simulink model "PMSM_SVPWM"  (R2021b)
settings: Solver=ode23tb  StartTime=0.0  StopTime=1  RelTol=1e-3  EnableMultiTasking=on
InitFcn:
  | flux=0.192;
  | Ld=0.0006033;
  | Lq=0.0006668;
  | R=0.05;
libraries: powerlib_extras x3, spsDCVoltageSourceLib x1, eeTransforms x1, spsPermanentMagnetSynchronousMachineLib x1, simulink x1, spsUniversalBridgeLib x1, spsVoltageMeasurementLib x1, spsdq0toabcLib x1, spspowerguiLib x1
settings Model: Creator=LZ  LastModifiedBy=wkw
settings SolverCC: AlgebraicLoopSolver=TrustRegion
settings DataIOCC: LimitDataPoints=on  SaveFormat=Array  ReturnWorkspaceOutputs=off
settings OptimizationCC: EfficientMapNaN2IntZero=off  LifeSpan=inf
settings DebuggingCC: SolverPrmCheckMsg=warning  SFUnexpectedBacktrackingDiag=warning  SFNoUnconditionalDefaultTransitionDiag=warning  SFMachineParentedDataDiag=warning  ArithmeticOperatorsInVariantConditions=warning
settings HardwareCC: ProdBitPerPointer=32  ProdBitPerSizeT=32  ProdBitPerPtrDiffT=32  ProdLargestAtomicFloat=None  ProdIntDivRoundTo=Undefined  ProdEndianess=Unspecified  ProdWordSize=32  ProdHWDeviceType=32-bit Generic  TargetBitPerLong=64  TargetBitPerPointer=64  TargetBitPerSizeT=64  TargetBitPerPtrDiffT=64  TargetLongLongMode=on  TargetIntDivRoundTo=Zero  TargetEndianess=LittleEndian  TargetWordSize=64  TargetHWDeviceType=MATLAB Host  ProdEqTarget=off
settings ModelReferenceCC: PropagateSignalLabelsOutOfModel=off
settings SFSimCC: SimUseLocalCustomCode=off  CustomCodeUndefinedFunction=UseInterfaceOnly
settings RTWCC: RTWUseLocalCustomCode=off
settings CodeAppCC: MaxIdLength=128  StateflowObjectComments=on
settings GRTTargetCC: TargetLangStandard=C89/C90 (ANSI)  CombineOutputUpdateFcns=off  GRTInterface=on
settings ConfigComp: CovMetricSettings=dw  CovSaveCumulativeToWorkspaceVar=on  CovSaveSingleToWorkspaceVar=on  CovExternalEMLEnable=off  CovSFcnEnable=off
settings SimscapeCC: SimscapeNormalizeSystem=off

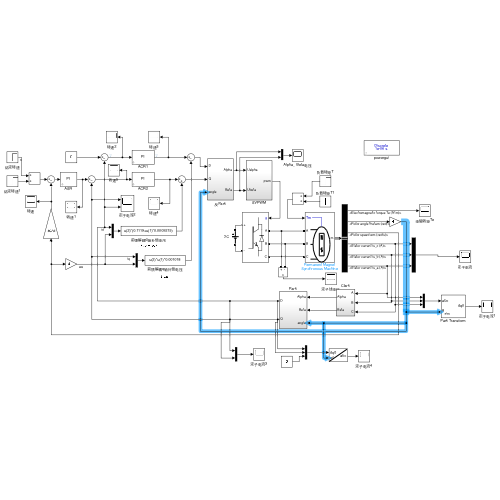
[thumbnail: Simulink's stored preview of the top-level diagram]
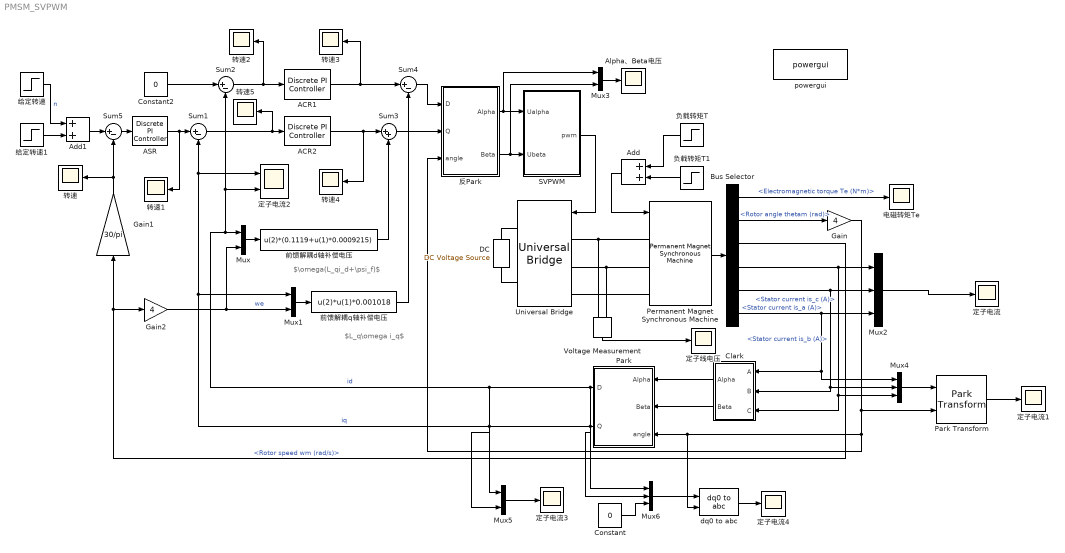
== system PMSM_SVPWM ==
  note: $\omega(L_qi_d+\psi_f)$
  note: $L_q\omega i_q$
  ACR1 : powerlib_extras/Discrete  Control Blocks/Discrete PI Controller  Kp=4  Ki=80  Par_Limits=[560*0.9*sqrt(1/3) -560*0.9*sqrt(1/3)]  Init=0  Ts=1e-6
  ACR2 : powerlib_extras/Discrete  Control Blocks/Discrete PI Controller  Kp=4  Ki=80  Par_Limits=[560*0.9*sqrt(1/3) -560*0.9*sqrt(1/3)]  Init=0  Ts=1e-6
  ASR : powerlib_extras/Discrete  Control Blocks/Discrete PI Controller  Kp=5  Ki=200  Par_Limits=[65 -65]  Init=0  Ts=1e-6
  Add : Sum
  Add1 : Sum
  Alpha、Beta电压 : Scope
  Bus Selector : BusSelector  OutputSignals=Electromagnetic torque Te (N*m),Rotor angle thetam (rad),Rotor speed wm (rad/s),Stator current is_c (A),Stator current is_b (A),Stator current is_a (A)
  Clark : Subsystem
  Constant : Constant  Value=0
  Constant2 : Constant  Value=0
  DC : spsDCVoltageSourceLib/DC Voltage Source  Amplitude=560  Measurements=None
  Gain : Gain  Gain=4
  Gain1 : Gain  Gain=30/pi
  Gain2 : Gain  Gain=4
  Mux{,1,3,5} (4 alike) : Mux  Inputs=2
  Mux2 : Mux  Inputs=3
  Mux4 : Mux  Inputs=3
  Mux6 : Mux  Inputs=3
  Park : Subsystem
  Park Transform : eeTransforms/Park Transform  AxisAlignment=D-axis  PowerInvariant=off
  Permanent Magnet Synchronous Machine : spsPermanentMagnetSynchronousMachineLib/Permanent Magnet Synchronous Machine  NbPhases=3  FluxDistribution=Sinusoidal  RotorType=Salient-pole  MechanicalLoad=Torque Tm  PresetModel=No  ShowDetailedParameters=on  MeasurementBus=off  Resistance=0.11  Inductance=8.5e-3  dqInductances=[0.0009215 0.001018]  La=0.000835  MachineConstant=Flux linkage established by magnets (V.s)  Flux=0.1119  VoltageCst=81.1857  TorqueCst=0.6714  Flat=120  Mechanical=[0.016 0.0002024 4 0]  PolePairs=4  InitialConditions=[0,0, 0,0]  InitialConditions5ph=[0 0 0 0 0 0]  RefAngle=Aligned with phase A axis (original Park)  IterativeDiscreteModel=Trapezoidal non iterative  TsBlock=-1  TsPowergui=0
  SVPWM : Subsystem
  Sum{1..2,4..5} (4 alike) : Sum  Inputs=|+-
  Sum3 : Sum  Inputs=|++
  Universal Bridge : spsUniversalBridgeLib/Universal Bridge  Arms=3  SnubberResistance=1e5  SnubberCapacitance=inf  Device=IGBT / Diodes  Ron=1e-3  Lon=0  ForwardVoltages="[  0  0  ]"  ForwardVoltage=0  GTOparameters=[ 10e-6 , 20e-6 ]  IGBTparameters=[ 1e-6 , 2e-6 ]  Measurements=None  Measurements_2=None  converterType=Rectifier
  Voltage Measurement : spsVoltageMeasurementLib/Voltage Measurement  PhasorSimulation=off  OutputType=Complex  PSBequivalent=0
  dq0 to abc : spsdq0toabcLib/dq0 to abc  Alignment=Aligned with phase A axis
  powergui : spspowerguiLib/powergui  Priority=1  SimulationMode=Discrete  SampleTime=1e-6  frequency=60  Iterations=50  frequencyindice=0  Pbase=100e6  ErrMax=1e-4  UnitsV=kV  UnitsW=MW  buscounter=0  FunctionMessages=off  echomessages=off  EnableUseOfTLC=off  CurrentSourceSwitches=off  DisableSnubberDevices=off  DisableRonSwitches=off  DisableVfSwitches=off  DisplayEquations=off  AutomaticDiscreteSolvers=off  SolverType=Tustin  Interpol=off  ExternalGateDelay=off  methode=off  Ts=0  x0status=blocks  SPID=off  SwTol=0  HookPort=off  NonlinearTolerance=1e-4  nMaxIteration=100  ContinueOnMaxIteration=off  RestoreLinks=warning  ResistiveCurrentMeasurement=off  Frange=[0:2:500]  Ylog=off  Xlog=on  ShowGrid=off  save=off  variable=ZData  structure=ScopeData7  ZoomFFT=on  StartTime=2.5  cycles=3  DisplayStyle=1  fundamental=60  FreqAxis=off  MaxFrequency=2000  frequencyindicesteady=1  RmsSteady=1  display=off
  前馈解耦d轴补偿电压 : Fcn  Expr=u(2)*(0.1119+u(1)*0.0009215)
  前馈解耦q轴补偿电压 : Fcn  Expr=u(2)*u(1)*0.001018
  反Park : Subsystem
  定子电流{,1,3..4} (4 alike) : Scope
  定子电流2 : Scope  NumInputPorts=2
  定子线电压 : Scope
  电磁转矩Te : Scope
  给定转速 : Step  Time=0  Before=1000  After=1000  SampleTime=0
  给定转速1 : Step  Time=0.7  After=200  SampleTime=0
  负载转矩T : Step  Time=0.5  After=20  SampleTime=0
  负载转矩T1 : Step  Time=0.03  After=0  SampleTime=0
  转速{,1..5} (6 alike) : Scope
  wires:
  Voltage Measurement/1 -> 定子线电压/1
  Permanent Magnet Synchronous Machine/1 -> Bus Selector/1
  Bus Selector/6 -> Mux2/3, Mux4/1, Clark/1(A)  "<Stator current is_a (A)>"
  Bus Selector/5 -> Mux2/2, Clark/2(B), Mux4/2  "<Stator current is_b (A)>"
  Bus Selector/4 -> Mux2/1, Clark/3(C), Mux4/3  "<Stator current is_c (A)>"
  SVPWM/1(pwm) -> Universal Bridge/1
  Clark/1(Alpha) -> Park/1(Alpha)
  Bus Selector/2 -> Gain/1  "<Rotor angle thetam (rad)>"
  Bus Selector/1 -> 电磁转矩Te/1  "<Electromagnetic torque Te (N*m)>"
  Bus Selector/3 -> Gain2/1, Gain1/1  "<Rotor speed wm (rad/s)>"
  Sum5/1 -> ASR/1
  Sum1/1 -> 转速5/1, ACR2/1
  Sum2/1 -> 转速2/1, ACR1/1
  Constant2/1 -> Sum2/1
  ACR1/1 -> 转速3/1, Sum4/1
  Park/1(D) -> Mux6/1, Mux5/1, 定子电流2/2, Sum2/2, Mux/1  "id"
  Park/2(Q) -> Mux6/2, Mux5/2, Mux1/1, 定子电流2/1, Sum1/2  "iq"
  Gain2/1 -> Mux1/2, Mux/2  "we"
  Mux/1 -> 前馈解耦d轴补偿电压/1
  Mux1/1 -> 前馈解耦q轴补偿电压/1
  Mux2/1 -> 定子电流/1
  Sum3/1 -> 反Park/2(Q)
  Sum4/1 -> 反Park/1(D)
  ACR2/1 -> 转速4/1, Sum3/1
  Clark/2(Beta) -> Park/2(Beta)
  给定转速/1 -> Add1/1  "n"
  反Park/1(Alpha) -> Mux3/1, SVPWM/1(Ualpha)
  反Park/2(Beta) -> Mux3/2, SVPWM/2(Ubeta)
  Mux3/1 -> Alpha、Beta电压/1
  负载转矩T/1 -> Add/1
  负载转矩T1/1 -> Add/2
  Add/1 -> Permanent Magnet Synchronous Machine/1
  Gain/1 -> Park Transform/2, 反Park/3(angle), dq0 to abc/2, Park/3(angle)
  ASR/1 -> 转速1/1, Sum1/1
  Gain1/1 -> 转速/1, Sum5/2
  前馈解耦d轴补偿电压/1 -> Sum3/2
  前馈解耦q轴补偿电压/1 -> Sum4/2
  给定转速1/1 -> Add1/2
  Add1/1 -> Sum5/1
  Mux4/1 -> Park Transform/1
  Park Transform/1 -> 定子电流1/1
  Mux5/1 -> 定子电流3/1
  Constant/1 -> Mux6/3
  Mux6/1 -> dq0 to abc/1
  dq0 to abc/1 -> 定子电流4/1
  connections:
  DC/RConn1 -- Universal Bridge/RConn1
  DC/LConn1 -- Universal Bridge/RConn2
  Voltage Measurement/LConn1 -- Permanent Magnet Synchronous Machine/LConn1 -- Universal Bridge/LConn1
  Voltage Measurement/LConn2 -- Permanent Magnet Synchronous Machine/LConn2 -- Universal Bridge/LConn2
  Permanent Magnet Synchronous Machine/LConn3 -- Universal Bridge/LConn3

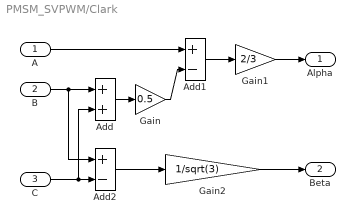
== system PMSM_SVPWM/Clark ==
  A : Inport
  B : Inport  Port=2
  C : Inport  Port=3
  Add : Sum
  Add1 : Sum  Inputs=+-
  Add2 : Sum  Inputs=+-
  Gain : Gain  Gain=0.5
  Gain1 : Gain  Gain=2/3
  Gain2 : Gain  Gain=1/sqrt(3)
  Alpha : Outport
  Beta : Outport  Port=2
  wires:
  B/1 -> Add2/1, Add/1
  C/1 -> Add/2, Add2/2
  Add/1 -> Gain/1
  A/1 -> Add1/1
  Gain/1 -> Add1/2
  Add1/1 -> Gain1/1
  Gain1/1 -> Alpha/1
  Add2/1 -> Gain2/1
  Gain2/1 -> Beta/1

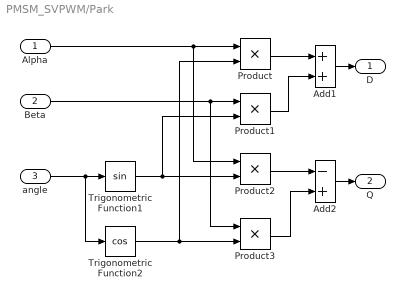
== system PMSM_SVPWM/Park ==
  Alpha : Inport
  Beta : Inport  Port=2
  angle : Inport  Port=3
  Add1 : Sum
  Add2 : Sum  Inputs=-+
  Product{,1..3} (4 alike) : Product
  Trigonometric Function1 : Trigonometry
  Trigonometric Function2 : Trigonometry  Operator=cos
  D : Outport
  Q : Outport  Port=2
  wires:
  Add2/1 -> Q/1
  Product3/1 -> Add2/2
  Product2/1 -> Add2/1
  Add1/1 -> D/1
  Product1/1 -> Add1/2
  Product/1 -> Add1/1
  Trigonometric Function1/1 -> Product2/2, Product1/2
  Beta/1 -> Product3/1, Product1/1
  Trigonometric Function2/1 -> Product3/2, Product/2
  Alpha/1 -> Product2/1, Product/1
  angle/1 -> Trigonometric Function1/1, Trigonometric Function2/1

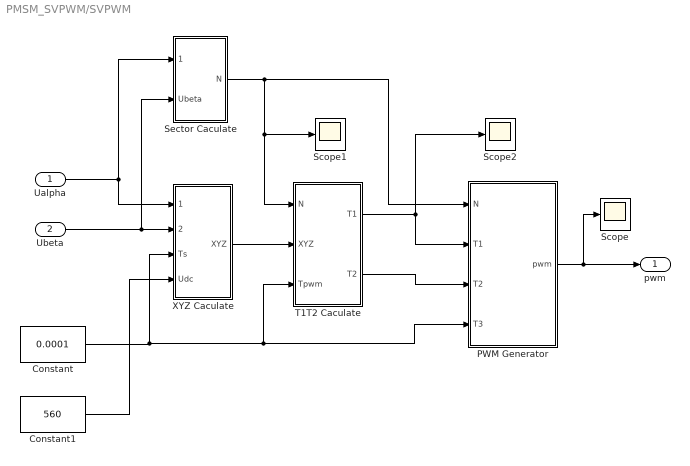
== system PMSM_SVPWM/SVPWM ==
  Ualpha : Inport
  Ubeta : Inport  Port=2
  Constant : Constant  Value=0.0001
  Constant1 : Constant  Value=560
  PWM Generator : Subsystem
  Scope : Scope
  Scope1 : Scope
  Scope2 : Scope
  Sector Caculate : Subsystem
  T1T2 Caculate : Subsystem
  XYZ Caculate : Subsystem
  pwm : Outport
  wires:
  Ualpha/1 -> XYZ Caculate/1(Ualpha), Sector Caculate/1(Ualpha)
  Ubeta/1 -> Sector Caculate/2("Ubeta "), XYZ Caculate/2(Ubeta)
  Constant/1 -> PWM Generator/4(T3), T1T2 Caculate/3(Tpwm), XYZ Caculate/3(Ts)
  Constant1/1 -> XYZ Caculate/4(Udc)
  XYZ Caculate/1(XYZ) -> T1T2 Caculate/2(XYZ)
  Sector Caculate/1(N) -> Scope1/1, T1T2 Caculate/1(N), PWM Generator/1(N)
  T1T2 Caculate/1("T1 ") -> PWM Generator/2(T1), Scope2/1
  T1T2 Caculate/2(T2) -> PWM Generator/3(T2)
  PWM Generator/1(pwm) -> pwm/1, Scope/1

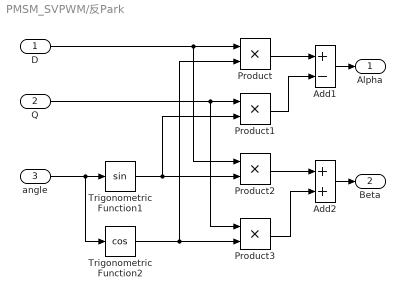
== system PMSM_SVPWM/反Park ==
  D : Inport
  Q : Inport  Port=2
  angle : Inport  Port=3
  Add1 : Sum  Inputs=+-
  Add2 : Sum
  Product{,1..3} (4 alike) : Product
  Trigonometric Function1 : Trigonometry
  Trigonometric Function2 : Trigonometry  Operator=cos
  Alpha : Outport
  Beta : Outport  Port=2
  wires:
  angle/1 -> Trigonometric Function2/1, Trigonometric Function1/1
  D/1 -> Product/1, Product2/1
  Trigonometric Function2/1 -> Product/2, Product3/2
  Q/1 -> Product1/1, Product3/1
  Trigonometric Function1/1 -> Product1/2, Product2/2
  Product/1 -> Add1/1
  Product1/1 -> Add1/2
  Add1/1 -> Alpha/1
  Product2/1 -> Add2/1
  Product3/1 -> Add2/2
  Add2/1 -> Beta/1

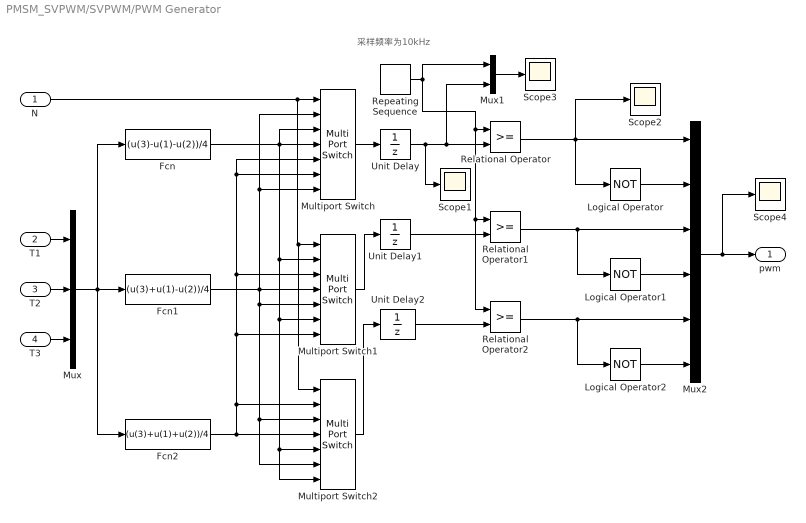
== system PMSM_SVPWM/SVPWM/PWM Generator ==
  note: 采样频率为10kHz
  N : Inport
  T1 : Inport  Port=2
  T2 : Inport  Port=3
  T3 : Inport  Port=4
  Fcn : Fcn  Expr=(u(3)-u(1)-u(2))/4
  Fcn1 : Fcn  Expr=(u(3)+u(1)-u(2))/4
  Fcn2 : Fcn  Expr=(u(3)+u(1)+u(2))/4
  Logical Operator : Logic  Operator=NOT  AllPortsSameDT=off  OutDataTypeStr=boolean
  Logical Operator1 : Logic  Operator=NOT  AllPortsSameDT=off  OutDataTypeStr=boolean
  Logical Operator2 : Logic  Operator=NOT  AllPortsSameDT=off  OutDataTypeStr=boolean
  Multiport Switch : MultiPortSwitch  Inputs=6  DiagnosticForDefault=None
  Multiport Switch1 : MultiPortSwitch  Inputs=6  DiagnosticForDefault=None
  Multiport Switch2 : MultiPortSwitch  Inputs=6  DiagnosticForDefault=None
  Mux : Mux  Inputs=3
  Mux1 : Mux  Inputs=2
  Mux2 : Mux  Inputs=6
  Relational Operator : RelationalOperator  OutDataTypeStr=boolean  RndMeth=Nearest
  Relational Operator1 : RelationalOperator  OutDataTypeStr=boolean  RndMeth=Nearest
  Relational Operator2 : RelationalOperator  OutDataTypeStr=boolean  RndMeth=Nearest
  Repeating Sequence : simulink/Sources/Repeating Sequence  rep_seq_t=[0 0.00005 0.0001]  rep_seq_y=[0 0.00005 0]
  Scope{1..4} (4 alike) : Scope
  Unit Delay : UnitDelay  SampleTime=0.0001  HasFrameUpgradeWarning=on
  Unit Delay1 : UnitDelay  SampleTime=0.0001  HasFrameUpgradeWarning=on
  Unit Delay2 : UnitDelay  SampleTime=0.0001  HasFrameUpgradeWarning=on
  pwm : Outport
  wires:
  T2/1 -> Mux/2
  T1/1 -> Mux/1
  T3/1 -> Mux/3
  Mux/1 -> Fcn/1, Fcn1/1, Fcn2/1
  N/1 -> Multiport Switch2/1, Multiport Switch1/1, Multiport Switch/1
  Fcn/1 -> Multiport Switch2/7, Multiport Switch2/5, Multiport Switch1/6, Multiport Switch1/2, Multiport Switch/4, Multiport Switch/3
  Fcn1/1 -> Multiport Switch/7, Multiport Switch/2, Multiport Switch2/6, Multiport Switch2/3, Multiport Switch1/5, Multiport Switch1/4
  Fcn2/1 -> Multiport Switch2/4, Multiport Switch2/2, Multiport Switch1/7, Multiport Switch1/3, Multiport Switch/6, Multiport Switch/5
  Repeating Sequence/1 -> Mux1/1, Relational Operator2/1, Relational Operator1/1, Relational Operator/1
  Relational Operator/1 -> Scope2/1, Logical Operator/1, Mux2/1
  Relational Operator1/1 -> Logical Operator1/1, Mux2/3
  Relational Operator2/1 -> Logical Operator2/1, Mux2/5
  Logical Operator/1 -> Mux2/2
  Logical Operator1/1 -> Mux2/4
  Logical Operator2/1 -> Mux2/6
  Mux2/1 -> Scope4/1, pwm/1
  Multiport Switch1/1 -> Unit Delay1/1
  Multiport Switch2/1 -> Unit Delay2/1
  Multiport Switch/1 -> Unit Delay/1
  Mux1/1 -> Scope3/1
  Unit Delay/1 -> Mux1/2, Relational Operator/2, Scope1/1
  Unit Delay1/1 -> Relational Operator1/2
  Unit Delay2/1 -> Relational Operator2/2

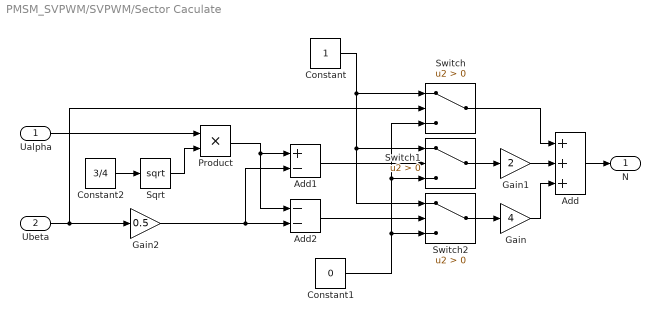
== system PMSM_SVPWM/SVPWM/Sector Caculate ==
  Ualpha : Inport
  "Ubeta " : Inport  Port=2
  Add : Sum  Inputs=+++
  Add1 : Sum  Inputs=+-
  Add2 : Sum  Inputs=--
  Constant : Constant
  Constant1 : Constant  Value=0
  Constant2 : Constant  Value=3/4
  Gain : Gain  Gain=4
  Gain1 : Gain  Gain=2
  Gain2 : Gain  Gain=0.5
  Product : Product
  Sqrt : Sqrt  SaturateOnIntegerOverflow=on
  Switch : Switch  Criteria=u2 > Threshold
  Switch1 : Switch  Criteria=u2 > Threshold
  Switch2 : Switch  Criteria=u2 > Threshold
  N : Outport
  wires:
  Ualpha/1 -> Product/1
  "Ubeta "/1 -> Switch/2, Gain2/1
  Add1/1 -> Switch1/2
  Add2/1 -> Switch2/2
  Constant/1 -> Switch/1, Switch1/1, Switch2/1
  Constant1/1 -> Switch2/3, Switch1/3, Switch/3
  Add/1 -> N/1
  Gain1/1 -> Add/2
  Gain/1 -> Add/3
  Switch2/1 -> Gain/1
  Switch1/1 -> Gain1/1
  Switch/1 -> Add/1
  Constant2/1 -> Sqrt/1
  Sqrt/1 -> Product/2
  Product/1 -> Add2/1, Add1/1
  Gain2/1 -> Add1/2, Add2/2

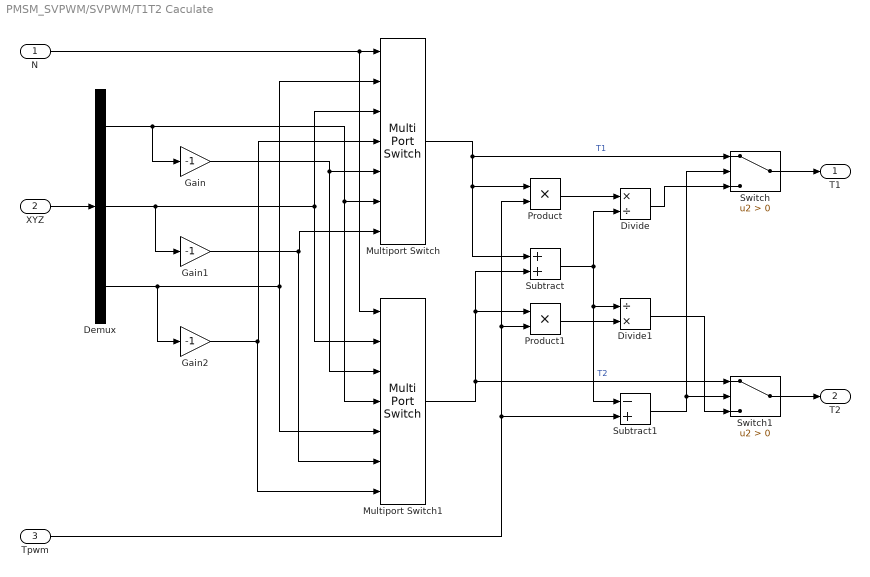
== system PMSM_SVPWM/SVPWM/T1T2 Caculate ==
  N : Inport
  XYZ : Inport  Port=2
  Tpwm : Inport  Port=3
  Demux : Demux  Outputs=3
  Divide : Product  Inputs=*/
  Divide1 : Product  Inputs=/*
  Gain : Gain  Gain=-1
  Gain1 : Gain  Gain=-1
  Gain2 : Gain  Gain=-1
  Multiport Switch : MultiPortSwitch  Inputs=6  DiagnosticForDefault=None
  Multiport Switch1 : MultiPortSwitch  Inputs=6  DiagnosticForDefault=None
  Product : Product
  Product1 : Product
  Subtract : Sum
  Subtract1 : Sum  Inputs=-+
  Switch : Switch  Criteria=u2 > Threshold
  Switch1 : Switch  Criteria=u2 > Threshold
  "T1 " : Outport
  T2 : Outport  Port=2
  wires:
  N/1 -> Multiport Switch1/1, Multiport Switch/1
  Demux/1 -> Multiport Switch1/4, Multiport Switch/6, Gain/1
  Demux/2 -> Multiport Switch/3, Multiport Switch1/2, Gain1/1
  Demux/3 -> Gain2/1, Multiport Switch1/5, Multiport Switch/2
  Gain/1 -> Multiport Switch/5, Multiport Switch1/3
  Gain1/1 -> Multiport Switch1/6, Multiport Switch/7
  Gain2/1 -> Multiport Switch1/7, Multiport Switch/4
  XYZ/1 -> Demux/1
  Multiport Switch/1 -> Switch/1, Product/1, Subtract/1  "T1"
  Multiport Switch1/1 -> Subtract/2, Product1/1, Switch1/1  "T2"
  Tpwm/1 -> Subtract1/2, Product/2, Product1/2
  Divide/1 -> Switch/3
  Divide1/1 -> Switch1/3
  Subtract1/1 -> Switch1/2, Switch/2
  Switch1/1 -> T2/1
  Switch/1 -> "T1 "/1
  Product/1 -> Divide/1
  Subtract/1 -> Divide/2, Divide1/1, Subtract1/1
  Product1/1 -> Divide1/2

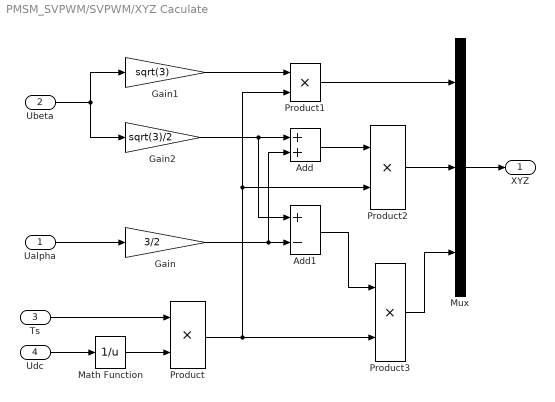
== system PMSM_SVPWM/SVPWM/XYZ Caculate ==
  Ualpha : Inport
  Ubeta : Inport  Port=2
  Ts : Inport  Port=3
  Udc : Inport  Port=4
  Add : Sum
  Add1 : Sum  Inputs=+-
  Gain : Gain  Gain=3/2
  Gain1 : Gain  Gain=sqrt(3)
  Gain2 : Gain  Gain=sqrt(3)/2
  Math Function : Math  Operator=reciprocal  SignedPower=on  SaturateOnIntegerOverflow=on
  Mux : Mux  Inputs=3
  Product{,1..3} (4 alike) : Product
  XYZ : Outport
  wires:
  Ualpha/1 -> Gain/1
  Ubeta/1 -> Gain2/1, Gain1/1
  Ts/1 -> Product/1
  Udc/1 -> Math Function/1
  Math Function/1 -> Product/2
  Gain1/1 -> Product1/1
  Product1/1 -> Mux/1
  Product/1 -> Product1/2, Product2/2, Product3/2
  Product3/1 -> Mux/3
  Gain/1 -> Add/2, Add1/2
  Gain2/1 -> Add1/1, Add/1
  Add/1 -> Product2/1
  Add1/1 -> Product3/1
  Product2/1 -> Mux/2
  Mux/1 -> XYZ/1
